simulink model "FunctionCall_Subsystem"  (R2021a)
settings: Solver=FixedStepAuto  StartTime=0.0  StopTime=10.0  FixedStep=1e-3  RelTol=1e-3
libraries: simulink x1
settings Model: Creator=lenovo  LastModifiedBy=lenovo

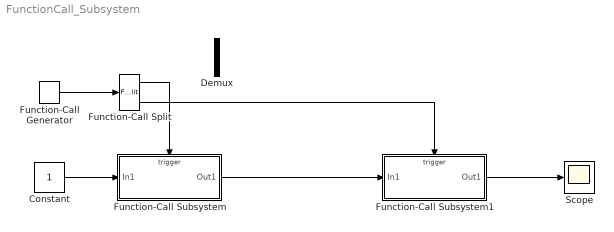
== system FunctionCall_Subsystem ==
  Constant : Constant
  Demux : Demux  Outputs=2
  Function-Call Generator : simulink/Ports & Subsystems/Function-Call Generator  sample_time=1  numberOfIterations=2  DisallowWideOutput=off
  Function-Call Split : FunctionCallSplit  IconShape=distinctive  NumOutputPorts=2  OutputPortLayout=default
  Function-Call Subsystem : Subsystem  TreatAsAtomicUnit=on
  Function-Call Subsystem1 : Subsystem  TreatAsAtomicUnit=on
  Scope : Scope
  wires:
  Constant/1 -> Function-Call Subsystem/1(In1)
  Function-Call Subsystem/1(Out1) -> Function-Call Subsystem1/1(In1)
  Function-Call Split/1 -> Function-Call Subsystem/Trigger
  Function-Call Split/2 -> Function-Call Subsystem1/Trigger
  Function-Call Subsystem1/1(Out1) -> Scope/1
  Function-Call Generator/1 -> Function-Call Split/1

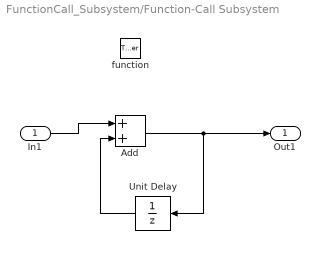
== system FunctionCall_Subsystem/Function-Call Subsystem ==
  In1 : Inport
  function : TriggerPort  TriggerType=function-call  VariantControl=(inherit)
  Add : Sum
  Unit Delay : UnitDelay  SampleTime=-1  HasFrameUpgradeWarning=on
  Out1 : Outport
  wires:
  Add/1 -> Unit Delay/1, Out1/1
  In1/1 -> Add/1
  Unit Delay/1 -> Add/2

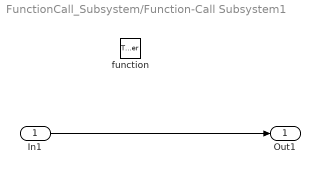
== system FunctionCall_Subsystem/Function-Call Subsystem1 ==
  In1 : Inport
  function : TriggerPort  TriggerType=function-call  VariantControl=(inherit)
  Out1 : Outport
  wires:
  In1/1 -> Out1/1
